simulink model "CubeSat_Simulator"  (R2019a)
settings: Solver=ode4  StartTime=0.0  StopTime=54000  FixedStep=0.1  RelTol=1e-5
model workspace: external: MATLAB File C:\Users\Heyang Zhang\OneDrive\02_Education\01_Undergraduate\02_Capstone\Killick-1 CubeSat\05_Technical\01_Simulation\01_Killick1\Simscape\Killick1_simScape_DataFile.m (data not in the file)
values from neighbouring files (symbols this model uses):
  a_desired = 0.35    [CubeSat_Parameter.m]
  D_distri = G_s.'* inv(G_s * G_s.')    [CubeSat_Parameter.m]
  G_s = [-cos(a_inc)*sin(b_rot)  -cos(a_inc)*cos(b_rot)   cos(a_inc)*sin(b_rot)  cos(a_inc)*cos(b_rot) ... (first row only)    [CubeSat_Parameter.m]
  I_rw = I_s - sum_rw    [CubeSat_Parameter.m]
  I_w = [3500E-9  3500E-9  3500E-9  3500E-9 ... (first row only)    [CubeSat_Parameter.m]
  Kc = [eye(3).*[2.5;2.5;2.5]  eye(3).*[5;5;5]]    [CubeSat_Parameter.m]
  Ki = [eye(3).*[1.2 1.2 1.2]  eye(3).*[3;3;3]]    [CubeSat_Parameter.m]
  Kw_d = 0.4    [CubeSat_Parameter.m]
  Kw_i = 0.1    [CubeSat_Parameter.m]
  Kw_p = 0.4    [CubeSat_Parameter.m]
  OMEGA_0 = [0;0;0]    [CubeSat_Parameter.m]
  quat_0 = eul2quat(eulr_0).'    [CubeSat_Parameter.m]
  SatMass = 3.5    [CubeSat_Parameter.m]
  tau_sat_mt = 1e-3    (= 0.001)    [CubeSat_Parameter.m]
  tau_sat_rw = 5e-3    (= 0.005)    [CubeSat_Parameter.m]
  w_desired = 0.35    [CubeSat_Parameter.m]
  w_rw_ref = [0;0;-0;-0]    [CubeSat_Parameter.m]
undefined symbols (not defined in the file or in its folder): Earth, IAU, km, Kp, Kv, s, WGS84
libraries: sharedutil x19, aerolibutil x18, dspmathops x18, sharedtransform x13, simulink_extras x8, aerolibtransform2 x5, simulink x5, asbCubeSatBlockLib x5, aerolibconvert2 x3, dsparch4 x3, ADCS_lib x2, aerolibcelestial x2
(part 2 of 3)

== system CubeSat_Simulator/CubeSat Hardware/Vehicle Dynamics/Orbital ==
  ExtForce_eci : Inport
  Gain : Gain  Gain=1/SatMass
  Initial Position : Constant  Value=[6778100;0;0]
  Initial Velocity : Constant  Value=[0;5444;5444]
  "Integrator, Second-Order" : SecondOrderIntegrator  ICSourceX=external  ICSourceDXDT=external
  Out Bus Element2 : Outport  PortName=SatStateOrbt  Element=x_eci
  Out Bus Element1 : Outport  PortName=SatStateOrbt  Element=v_eci
  Out Bus Element3 : Outport  PortName=SatStateOrbt  Element=a_eci
  wires:
  Gain/1 -> Out Bus Element3/1, "Integrator, Second-Order"/1
  ExtForce_eci/1 -> Gain/1
  "Integrator, Second-Order"/1 -> Out Bus Element2/1
  "Integrator, Second-Order"/2 -> Out Bus Element1/1
  Initial Velocity/1 -> "Integrator, Second-Order"/3
  Initial Position/1 -> "Integrator, Second-Order"/2

== system CubeSat_Simulator/Environment/Earth Rotation Planet Position/Celestrial Body Position ==
  JulianDate : Inport
  Length Conversion : aerolibconvert2/Length Conversion  IU=km  OU=m
  Length Conversion1 : aerolibconvert2/Length Conversion  IU=km  OU=m
  Moon Position_ECI : aerolibcelestial/Planetary Ephemeris  kmflag=km,km/s  epochflag=Julian date  de=DE405  nCenter=Earth  nTarget=Moon  errorflag=Error  velflag=off
      settings: SourceProductName=Aerospace Blockset  SourceProductBaseCode=AE
  Sun Position_ECI : aerolibcelestial/Planetary Ephemeris  kmflag=km,km/s  epochflag=Julian date  de=DE405  nCenter=Earth  nTarget=Sun  errorflag=Error  velflag=off
      settings: SourceProductName=Aerospace Blockset  SourceProductBaseCode=AE
  x_sun_eci : Outport
  x_moon_eci : Outport  Port=2
  wires:
  Sun Position_ECI/1 -> Length Conversion/1
  JulianDate/1 -> Moon Position_ECI/1, Sun Position_ECI/1
  Moon Position_ECI/1 -> Length Conversion1/1
  Length Conversion/1 -> x_sun_eci/1  "x_sun_eci"
  Length Conversion1/1 -> x_moon_eci/1  "x_moon_eci"

== system CubeSat_Simulator/Environment/Earth Rotation Planet Position/Earth Rotation  ==
  SimTime : Inport
  Direction Cosine Matrix to Quaternions : sharedtransform/Direction Cosine Matrix  to Quaternions  aMode=0  action=None  tolerance=eps(2)
      settings: SourceProductName=Aerospace Blockset  SourceProductBaseCode=AE
  Direction Cosine Matrix to Quaternions1 : sharedtransform/Direction Cosine Matrix  to Quaternions  aMode=0  action=None  tolerance=eps(2)
      settings: SourceProductName=Aerospace Blockset  SourceProductBaseCode=AE
  ECI to ECEF DCM : aerolibtransform2/Direction Cosine Matrix ECI to ECEF  red=IAU-2000/2006  year=2019  month=July  day=1  hour=0  min=0  sec=0  deltaT=Sec  errorflag=Error  extraparamflag=off
      settings: AttributesFormatString=%<red>  SourceProductName=Aerospace Blockset  SourceProductBaseCode=AE
  Transpose : Math  Operator=transpose  SaturateOnIntegerOverflow=on
  q_eci2ecef : Outport
  q_ecef2eci : Outport  Port=2
  wires:
  Transpose/1 -> Direction Cosine Matrix to Quaternions1/1
  Direction Cosine Matrix to Quaternions1/1 -> q_ecef2eci/1
  Direction Cosine Matrix to Quaternions/1 -> q_eci2ecef/1
  ECI to ECEF DCM/1 -> Direction Cosine Matrix to Quaternions/1, Transpose/1
  SimTime/1 -> ECI to ECEF DCM/1

== system CubeSat_Simulator/Environment/External Force and Torque/Earth Gravity Pull ==
  x_ecef : Inport
  Gain : Gain  Gain=SatMass
  Spherical Harmonic Gravity Model : aerolibgravity2/Spherical Harmonic Gravity Model  units=Metric (MKS)  degree=120  action=Warning  ptype=EGM2008  datafile='aerogmm2b.mat'
      settings: SourceProductName=Aerospace Blockset  SourceProductBaseCode=AE
  f_grav_ecef : Outport
  wires:
  Spherical Harmonic Gravity Model/1 -> Gain/1
  Gain/1 -> f_grav_ecef/1
  x_ecef/1 -> Spherical Harmonic Gravity Model/1

== system CubeSat_Simulator/Environment/External Force and Torque/Exp Decay Air Density ==
  h (m) : Inport
  2-D Lookup Table : Lookup_n-D  BreakpointsForDimension1=[12.5 27.5:5:97.5 105:10:170 190 225:50:475 550:100:950]  BreakpointsForDimension2=[1:3]  Table=[0 1.225 8.44; 25 3.899e-2 6.49; 30 1.774e-2 6.75; 35 8.279e-3 7.07; 40 3.972e-3 7.47; 45 1.995e-3 7.83; 50 1.057e-3 7.95; 55 5.821e-4 7.73; 60 3.206e-4 7.29; 65 1.718e-4 6.81; 70 8.770e-5 6.33; 75 4.178e-5 6; 80 1.905e-5 5.7; 85 8.337e-6 5.41; 90 3.396e-6 5.38; 95 1.343e-6 5.74; 100 5.297e-7 6.15; 110 9.661e-8 8.06; 120 2.438e-8 11.6; 130 8.484e-9 16.1; 140 3.845e-9 20.6; 150 2.07e-9 24.6; 160 1.224e-9 26.3; 180 5.464e-10 33.2; 200 2.789e-10 38.5; 250 7.248e-11 46.9; 300 2.418e-11 52.5; 350 9.158e-12 56.4; 400 3.725e-12 59.4; 450 1.585e-12 62.2; 500 6.967e-13 65.8; 600 1.454e-13 79; 700 3.614e-14 109; 800 1.17e-14 164; 900 5.245e-15 225]  InternalRulePriority=Speed  RndMeth=Simplest  InputSameDT=on
  2-D Lookup Table1 : Lookup_n-D  BreakpointsForDimension1=[12.5 27.5:5:97.5 105:10:170 190 225:50:475 550:100:950]  BreakpointsForDimension2=[1:3]  Table=[0 1.225 8.44; 25 3.899e-2 6.49; 30 1.774e-2 6.75; 35 8.279e-3 7.07; 40 3.972e-3 7.47; 45 1.995e-3 7.83; 50 1.057e-3 7.95; 55 5.821e-4 7.73; 60 3.206e-4 7.29; 65 1.718e-4 6.81; 70 8.770e-5 6.33; 75 4.178e-5 6; 80 1.905e-5 5.7; 85 8.337e-6 5.41; 90 3.396e-6 5.38; 95 1.343e-6 5.74; 100 5.297e-7 6.15; 110 9.661e-8 8.06; 120 2.438e-8 11.6; 130 8.484e-9 16.1; 140 3.845e-9 20.6; 150 2.07e-9 24.6; 160 1.224e-9 26.3; 180 5.464e-10 33.2; 200 2.789e-10 38.5; 250 7.248e-11 46.9; 300 2.418e-11 52.5; 350 9.158e-12 56.4; 400 3.725e-12 59.4; 450 1.585e-12 62.2; 500 6.967e-13 65.8; 600 1.454e-13 79; 700 3.614e-14 109; 800 1.17e-14 164; 900 5.245e-15 225]  InternalRulePriority=Speed  RndMeth=Simplest  InputSameDT=on
  2-D Lookup Table2 : Lookup_n-D  BreakpointsForDimension1=[12.5 27.5:5:97.5 105:10:170 190 225:50:475 550:100:950]  BreakpointsForDimension2=[1:3]  Table=[0 1.225 8.44; 25 3.899e-2 6.49; 30 1.774e-2 6.75; 35 8.279e-3 7.07; 40 3.972e-3 7.47; 45 1.995e-3 7.83; 50 1.057e-3 7.95; 55 5.821e-4 7.73; 60 3.206e-4 7.29; 65 1.718e-4 6.81; 70 8.770e-5 6.33; 75 4.178e-5 6; 80 1.905e-5 5.7; 85 8.337e-6 5.41; 90 3.396e-6 5.38; 95 1.343e-6 5.74; 100 5.297e-7 6.15; 110 9.661e-8 8.06; 120 2.438e-8 11.6; 130 8.484e-9 16.1; 140 3.845e-9 20.6; 150 2.07e-9 24.6; 160 1.224e-9 26.3; 180 5.464e-10 33.2; 200 2.789e-10 38.5; 250 7.248e-11 46.9; 300 2.418e-11 52.5; 350 9.158e-12 56.4; 400 3.725e-12 59.4; 450 1.585e-12 62.2; 500 6.967e-13 65.8; 600 1.454e-13 79; 700 3.614e-14 109; 800 1.17e-14 164; 900 5.245e-15 225]  InternalRulePriority=Speed  RndMeth=Simplest  InputSameDT=on
  Index: H [km] : Constant  Value=3
  Index: h_0 [km] : Constant
  Index: rho_0 [kg/m3] : Constant  Value=2
  MATLAB Function3 : MATLAB Function  TreatAsAtomicUnit=on
  Multiply : Gain  Gain=1/1000
  rho (kg/m3) : Outport
  wires:
  Multiply/1 -> 2-D Lookup Table1/1, 2-D Lookup Table/1, 2-D Lookup Table2/1, MATLAB Function3/1(h)
  2-D Lookup Table/1 -> MATLAB Function3/2(h_0)
  2-D Lookup Table2/1 -> MATLAB Function3/4(H)
  Index: rho_0 [kg/m3]/1 -> 2-D Lookup Table1/2
  2-D Lookup Table1/1 -> MATLAB Function3/3(rho_0)
  h (m)/1 -> Multiply/1
  Index: h_0 [km]/1 -> 2-D Lookup Table/2
  Index: H [km]/1 -> 2-D Lookup Table2/2
  MATLAB Function3/1(rho) -> rho (kg/m3)/1

== system CubeSat_Simulator/Environment/External Force and Torque/q to w ==
  q : Inport
  Derivative : Derivative
  Product : Product
  Quaternion to Spatial Rotation : Subsystem
  w : Outport
  wires:
  q/1 -> Quaternion to Spatial Rotation/1(q)
  Derivative/1 -> Product/1
  Product/1 -> w/1
  Quaternion to Spatial Rotation/1(PRA) -> Derivative/1
  Quaternion to Spatial Rotation/2(PRV) -> Product/2  "ehat"

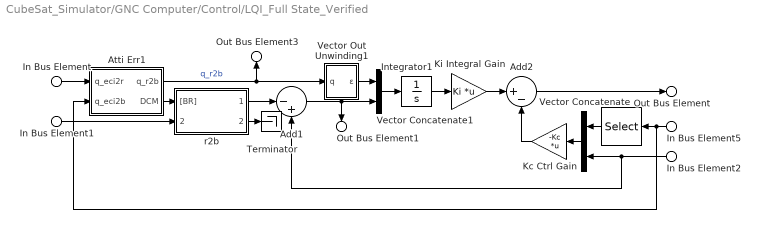
== system CubeSat_Simulator/GNC Computer/Control/LQI_Full State_Verified ==
  In Bus Element : Inport  PortName=GdnIn  Element=q_eci2ref
  In Bus Element1 : Inport  PortName=GdnIn  Element=r_w_r/n
  In Bus Element5 : Inport  Port=2  PortName=NavIn  Element=q_eci2body
  In Bus Element2 : Inport  Port=2  PortName=NavIn  Element=b_w_b/n
  " " : Selector  InputPortWidth=4  IndexOptions=Index vector (dialog)  Indices=[2 3 4]  OutputSizes=1
  Add1 : Sum  Inputs=|-+
  Add2 : Sum  Inputs=|+-
  Atti Err1 : Subsystem
  Integrator1 : Integrator
  Kc Ctrl Gain : Gain  Gain=-Kc  Multiplication=Matrix(K*u)
  Ki Integral Gain : Gain  Gain=Ki  Multiplication=Matrix(K*u)
  Terminator : Terminator
  Vector Concatenate : Concatenate
  Vector Concatenate1 : Concatenate
  Vector Out Unwinding1 : Subsystem
  r2b : Subsystem
  Out Bus Element : Outport  PortName=ACCmd  Element=b_t_total
  Out Bus Element3 : Outport  Port=2  PortName=ErrData  Element=q_r2b
  Out Bus Element1 : Outport  Port=2  PortName=ErrData  Element=deltaw_b/r
  wires:
  Vector Concatenate1/1 -> Integrator1/1
  Vector Out Unwinding1/1(ε) -> Vector Concatenate1/1
  Vector Concatenate/1 -> Kc Ctrl Gain/1
  " "/1 -> Vector Concatenate/1
  Integrator1/1 -> Ki Integral Gain/1
  Add2/1 -> Out Bus Element/1
  Kc Ctrl Gain/1 -> Add2/2
  Ki Integral Gain/1 -> Add2/1
  r2b/2(b_a_r/n) -> Terminator/1
  r2b/1(b_w_r/n) -> Add1/1
  In Bus Element2/1 -> Add1/2, Vector Concatenate/2
  In Bus Element/1 -> Atti Err1/1(q_eci2r)
  Atti Err1/2(DCM) -> r2b/1("[BR]")
  In Bus Element5/1 -> Atti Err1/2(q_eci2b), " "/1
  Atti Err1/1(q_r2b) -> Vector Out Unwinding1/1(q), Out Bus Element3/1  "q_r2b"
  Add1/1 -> Vector Concatenate1/2, Out Bus Element1/1
  In Bus Element1/1 -> r2b/2(r_w_r/n)

== system CubeSat_Simulator/GNC Computer/Control/Momentum Management1 ==
  ACCmd : Inport
  w_rw : Inport  Port=2
  Add : Sum  Inputs=|++
  Bus Creator : BusCreator  Inputs=2
  G_s : Gain  Gain=G_s  Multiplication=Matrix(K*u)
  de-spin torq : Subsystem
  Out Bus Element : Outport  PortName=MMCmd  Element=MMTorqCmd
  wires:
  Bus Creator/1 -> Out Bus Element/1
  ACCmd/1 -> Add/1
  G_s/1 -> Add/2, Bus Creator/2  "b_t_cmd_mtc"
  Add/1 -> Bus Creator/1  "b_t_cmd_rwc"
  w_rw/1 -> de-spin torq/1(w_rw)
  de-spin torq/1(u_despin) -> G_s/1

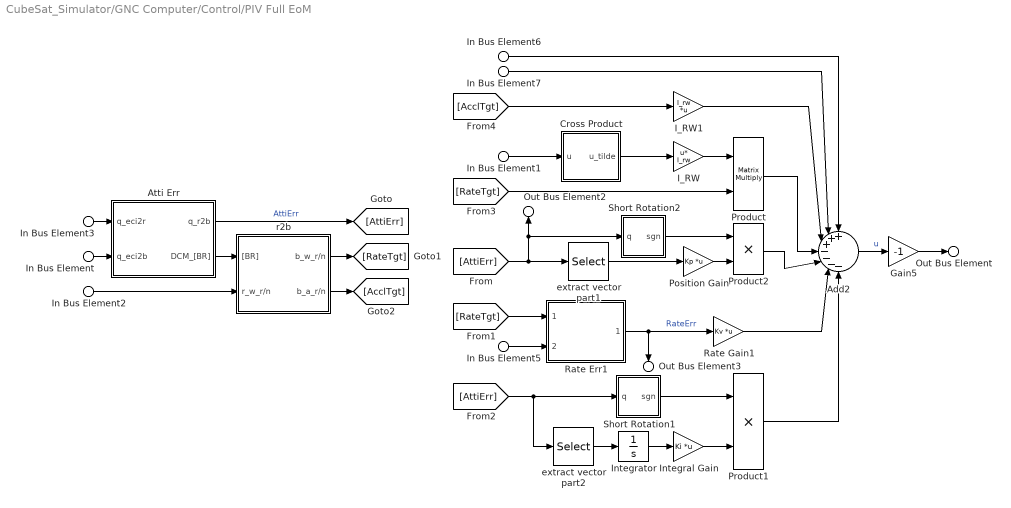
== system CubeSat_Simulator/GNC Computer/Control/PIV Full EoM ==
  In Bus Element3 : Inport  PortName=GdnIn  Element=q_eci2ref
  In Bus Element2 : Inport  PortName=GdnIn  Element=r_w_r/n
  In Bus Element : Inport  Port=2  PortName=NavIn  Element=q_eci2body
  In Bus Element5 : Inport  Port=2  PortName=NavIn  Element=b_w_b/n
  In Bus Element1 : Inport  Port=2  PortName=NavIn  Element=b_w_b/n
  In Bus Element6 : Inport  Port=2  PortName=NavIn  Element=gyroscopic
  In Bus Element7 : Inport  Port=2  PortName=NavIn  Element=momentum
  Add2 : Sum  Inputs=+++----
  Atti Err : Subsystem
  Cross Product : MATLAB Function  TreatAsAtomicUnit=on
  Gain5 : Gain  Gain=-1
  I_RW : Gain  Gain=I_rw  Multiplication=Matrix(u*K)
  I_RW1 : Gain  Gain=I_rw  Multiplication=Matrix(K*u)
  Integral Gain : Gain  Gain=Ki  Multiplication=Matrix(K*u)
  Integrator : Integrator
  Position Gain : Gain  Gain=Kp  Multiplication=Matrix(K*u)
  Product : Product  Multiplication=Matrix(*)
  Product1 : Product
  Product2 : Product
  Rate Err1 : Subsystem
  Rate Gain1 : Gain  Gain=Kv  Multiplication=Matrix(K*u)
  Short Rotation1 : Subsystem
  Short Rotation2 : Subsystem
  extract vector part1 : Selector  InputPortWidth=4  IndexOptions=Index vector (dialog)  Indices=[2 3 4]  OutputSizes=1
  extract vector part2 : Selector  InputPortWidth=4  IndexOptions=Index vector (dialog)  Indices=[2 3 4]  OutputSizes=1
  r2b : Subsystem
  Out Bus Element : Outport  PortName=ACCmd  Element=b_t_total
  Out Bus Element3 : Outport  Port=2  PortName=ErrData  Element=deltaw_b/r
  Out Bus Element2 : Outport  Port=2  PortName=ErrData  Element=q_r2b
  wires:
  Rate Gain1/1 -> Add2/6
  In Bus Element6/1 -> Add2/1
  In Bus Element7/1 -> Add2/2
  I_RW1/1 -> Add2/3
  Product/1 -> Add2/4
  Product2/1 -> Add2/5
  Product1/1 -> Add2/7
  [AcclTgt] -> I_RW1/1
  [RateTgt] -> Product/2
  extract vector part1/1 -> Position Gain/1
  [AttiErr] -> extract vector part1/1, Out Bus Element2/1, Short Rotation2/1(q)
  Short Rotation2/1(sgn) -> Product2/1
  Position Gain/1 -> Product2/2
  Atti Err/1(q_r2b) -> [AttiErr]  "AttiErr"
  In Bus Element2/1 -> r2b/2(r_w_r/n)
  r2b/2(b_a_r/n) -> [AcclTgt]
  Add2/1 -> Gain5/1  "u"
  Gain5/1 -> Out Bus Element/1
  Rate Err1/1(b_deltaw_b/r) -> Out Bus Element3/1, Rate Gain1/1  "RateErr"
  In Bus Element5/1 -> Rate Err1/2(b_w_b/n)
  In Bus Element3/1 -> Atti Err/1(q_eci2r)
  r2b/1(b_w_r/n) -> [RateTgt]
  Atti Err/2(DCM_[BR]) -> r2b/1("[BR]")
  Integral Gain/1 -> Product1/2
  Short Rotation1/1(sgn) -> Product1/1
  [AttiErr] -> extract vector part2/1, Short Rotation1/1(q)
  Integrator/1 -> Integral Gain/1
  extract vector part2/1 -> Integrator/1
  [RateTgt] -> Rate Err1/1(b_w_r/n)
  Cross Product/1(u_tilde) -> I_RW/1
  In Bus Element1/1 -> Cross Product/1(u)
  I_RW/1 -> Product/1
  In Bus Element/1 -> Atti Err/2(q_eci2b)

== system CubeSat_Simulator/GNC Computer/Guidance/Inertial Pointing ==
  Degrees to Radians : simulink_extras/Transformations/Degrees to Radians
  Spatial Rotation to Quaternion : Subsystem
  Step1 : Step  Time=10  After=0  SampleTime=0
  axis : Constant  Value=[1;1;1]
  q_eci2iner : Outport
  wires:
  axis/1 -> Spatial Rotation to Quaternion/2(PRV)
  Degrees to Radians/1 -> Spatial Rotation to Quaternion/1(PRA)
  Step1/1 -> Degrees to Radians/1
  Spatial Rotation to Quaternion/1(q) -> q_eci2iner/1

== system CubeSat_Simulator/GNC Computer/Guidance/Nadir Pointing ==
  NadirBias : Inport
  SensorIn : Inport  Port=2
  Align Body Axis : Subsystem
  Apply Orientation Bias : Subsystem
  Calculate Hill Frame : Subsystem
  q_eci2nadr : Outport
  wires:
  Align Body Axis/1(q_eci2ndir) -> Apply Orientation Bias/1(q_eci2ndir)
  Apply Orientation Bias/1(q_eci2imag) -> q_eci2nadr/1
  NadirBias/1 -> Apply Orientation Bias/2(NadirBias)
  SensorIn/1 -> Calculate Hill Frame/1(SensorIn)
  Calculate Hill Frame/1(q_eci2hill) -> Align Body Axis/1(q_eci2hill)

== system CubeSat_Simulator/GNC Computer/Guidance/Orbital Velocity Frame (Visualization Only) ==
  In Bus Element1 : Inport  PortName=SensorIn  Element=x_eci
  In Bus Element2 : Inport  PortName=SensorIn  Element=v_eci
  3x3 Cross Product2 : sharedutil/3x3 Cross Product  aMode=aMode
      settings: SourceProductBaseCode=AE
  3x3 Cross Product3 : sharedutil/3x3 Cross Product  aMode=aMode
      settings: SourceProductBaseCode=AE
  Direction Cosine Matrix to Quaternions : sharedtransform/Direction Cosine Matrix  to Quaternions  aMode=0  action=None  tolerance=eps(2)
      settings: SourceProductName=Aerospace Blockset  SourceProductBaseCode=AE
  Gain : Gain  Gain=-1
  Normalization3 : dspmathops/Normalization  NormType=2-norm  Bias=1e-10  NormOver=Each column  Dimension=1  roundingMode=Floor  overflowMode=off  accumDataTypeStr=Inherit: Same as product output  accumLastDataTypeStr=Inherit: Same as product output  outputDataTypeStr=Inherit: Same as product output  outputMin=[]  outputMax=[]  outputLastDataTypeStr=Inherit: Same as product output
      settings: SourceProductName=DSP System Toolbox
  Normalization4 : dspmathops/Normalization  NormType=2-norm  Bias=1e-10  NormOver=Each column  Dimension=1  roundingMode=Floor  overflowMode=off  accumDataTypeStr=Inherit: Same as product output  accumLastDataTypeStr=Inherit: Same as product output  outputDataTypeStr=Inherit: Same as product output  outputMin=[]  outputMax=[]  outputLastDataTypeStr=Inherit: Same as product output
      settings: SourceProductName=DSP System Toolbox
  Quaternion Normalize : sharedutil/Quaternion Normalize  aMode=aMode
      settings: SourceProductName=Aerospace Blockset  SourceProductBaseCode=AE
  Transpose : Math  Operator=transpose  SaturateOnIntegerOverflow=on
  Transpose1 : Math  Operator=transpose  SaturateOnIntegerOverflow=on
  Transpose2 : Math  Operator=transpose  SaturateOnIntegerOverflow=on
  Vector Concatenate : Concatenate  NumInputs=3  Mode=Multidimensional array
  q_eci2velo : Outport
  wires:
  Direction Cosine Matrix to Quaternions/1 -> Quaternion Normalize/1
  Transpose1/1 -> Vector Concatenate/3
  Vector Concatenate/1 -> Direction Cosine Matrix to Quaternions/1
  Transpose2/1 -> Vector Concatenate/2
  Transpose/1 -> Vector Concatenate/1
  In Bus Element2/1 -> Normalization3/1
  Normalization3/1 -> Gain/1
  Gain/1 -> 3x3 Cross Product3/1, Transpose/1, 3x3 Cross Product2/2
  In Bus Element1/1 -> Normalization4/1
  Normalization4/1 -> 3x3 Cross Product2/1
  3x3 Cross Product2/1 -> Transpose2/1, 3x3 Cross Product3/2
  3x3 Cross Product3/1 -> Transpose1/1
  Quaternion Normalize/1 -> q_eci2velo/1

== system CubeSat_Simulator/GNC Computer/Guidance/Sun Tracking ==
  SunBias : Inport
  In Bus Element1 : Inport  Port=2  PortName=SensorIn  Element=x_eci
  In Bus Element : Inport  Port=3  PortName=EnvState  Element=Celestrial.x_sun_eci
  Add1 : Sum  Inputs=+-
  Attitude Bias : Subsystem
  Check Parallel : asbCubeSatBlockLib/Axes Transformations/Attitude Conversion/Check Parallel  SystemSampleTime=-1
  Compare To Zero1 : simulink/Logic and Bit Operations/Compare To Zero  relop=~=  OutDataTypeStr=boolean
  Compute Sun Frame : Subsystem
  ECI X Axis : Constant  Value=[1;0;0]
  ECI Z Axis : Constant  Value=[0;0;1]
  If Sun Directly Above ECI : asbCubeSatBlockLib/Axes Transformations/Attitude Conversion/Quaternion between r_a and r_b  SystemSampleTime=-1
  Switch 1 走上 0 走下 : Switch  Criteria=u2 ~= 0
  q_eci2sun : Outport
  wires:
  Add1/1 -> If Sun Directly Above ECI/2, Check Parallel/1, Compute Sun Frame/1(FirstRefECI)
  ECI Z Axis/1 -> Check Parallel/2, Compute Sun Frame/2(SecondRefECI)
  Compute Sun Frame/1(q_eci2sun) -> Switch 1 走上 0 走下/3
  In Bus Element/1 -> Add1/1
  In Bus Element1/1 -> Add1/2
  ECI X Axis/1 -> If Sun Directly Above ECI/1
  If Sun Directly Above ECI/1 -> Switch 1 走上 0 走下/1
  Check Parallel/1 -> Compare To Zero1/1
  Compare To Zero1/1 -> Switch 1 走上 0 走下/2
  Switch 1 走上 0 走下/1 -> Attitude Bias/1(q Input)
  Attitude Bias/1("\tq Output") -> q_eci2sun/1
  SunBias/1 -> Attitude Bias/2(EulerBias)

== system CubeSat_Simulator/GNC Computer/Guidance/Target Tracking ==
  TargetLLA : Inport
  TargetBias : Inport  Port=2
  In Bus Element1 : Inport  Port=3  PortName=SensorIn  Element=x_eci
  In Bus Element : Inport  Port=4  PortName=EnvState  Element=Celestrial.q_ecef2eci
  Add1 : Sum  Inputs=|+-
  Attitude Bias : Subsystem
  Check Parallel : asbCubeSatBlockLib/Axes Transformations/Attitude Conversion/Check Parallel  SystemSampleTime=-1
  Compare To Zero1 : simulink/Logic and Bit Operations/Compare To Zero  relop=~=  OutDataTypeStr=boolean
  Compute Sun Frame : Subsystem
  Demux : Demux  Outputs=3
  ECI X Axis : Constant  Value=[1;0;0]
  ECI Z Axis : Constant  Value=[0;0;1]
  If Sun Directly Above ECI : asbCubeSatBlockLib/Axes Transformations/Attitude Conversion/Quaternion between r_a and r_b  SystemSampleTime=-1
  "LLA to ECEF Position " : aerolibtransform2/LLA to ECEF Position  units=Metric (MKS)  ptype=Earth (WGS84)  F=1/298.257223563  R=6378137
      settings: SourceProductName=Aerospace Blockset  SourceProductBaseCode=AE
  Mux : Mux  Inputs=2
  Switch 1 走上 0 走下 : Switch  Criteria=u2 ~= 0
  Target Position ECEF to ECI : aerolibutil/Quaternion Rotation
  q_eci2lla : Outport
  tag scope: TgtPos_eci=global
  wires:
  Attitude Bias/1("\tq Output") -> q_eci2lla/1
  In Bus Element/1 -> Target Position ECEF to ECI/1
  "LLA to ECEF Position "/1 -> Target Position ECEF to ECI/2
  Demux/1 -> Mux/1
  Demux/2 -> Mux/2
  Mux/1 -> "LLA to ECEF Position "/1
  TargetLLA/1 -> Demux/1
  Demux/3 -> "LLA to ECEF Position "/2
  In Bus Element1/1 -> Add1/1
  Target Position ECEF to ECI/1 -> Add1/2
  Add1/1 -> Compute Sun Frame/1(FirstRefECI), [TgtPos_eci], Check Parallel/1, If Sun Directly Above ECI/2  "TgtPos_eci"
  If Sun Directly Above ECI/1 -> Switch 1 走上 0 走下/1
  TargetBias/1 -> Attitude Bias/2(EulerBias)
  Check Parallel/1 -> Compare To Zero1/1
  Switch 1 走上 0 走下/1 -> Attitude Bias/1(q Input)
  ECI X Axis/1 -> If Sun Directly Above ECI/1
  Compare To Zero1/1 -> Switch 1 走上 0 走下/2
  ECI Z Axis/1 -> Check Parallel/2, Compute Sun Frame/2(SecondRefECI)
  Compute Sun Frame/1(q_eci2sun) -> Switch 1 走上 0 走下/3

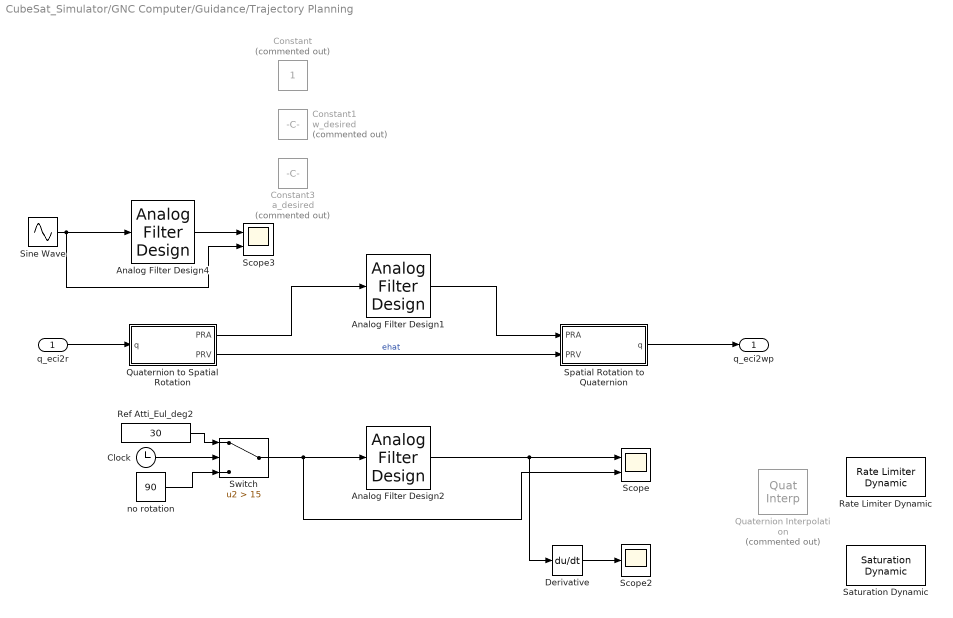
== system CubeSat_Simulator/GNC Computer/Guidance/Trajectory Planning ==
  q_eci2r : Inport
  Analog Filter Design1 : dsparch4/Analog Filter Design  method=Bessel  filttype=Lowpass  N=10  Wlo=0.1  Whi=80  Rp=2  Rs=40
  Analog Filter Design2 : dsparch4/Analog Filter Design  method=Bessel  filttype=Lowpass  N=10  Wlo=0.5  Whi=80  Rp=2  Rs=40
  Analog Filter Design4 : dsparch4/Analog Filter Design  method=Bessel  filttype=Lowpass  N=10  Wlo=0.1  Whi=80  Rp=2  Rs=40
  Clock : Clock
  Constant : Constant  Commented=on
  Constant1 : Constant  Commented=on  Value=w_desired
  Constant3 : Constant  Commented=on  Value=a_desired
  Derivative : Derivative
  Quaternion Interpolation : QuatInterp  Commented=on
  Quaternion to Spatial Rotation : Subsystem
  Rate Limiter Dynamic : simulink/Discontinuities/Rate Limiter Dynamic
      settings: SourceProductName=Simulink
  Ref Atti_Eul_deg2 : Constant  Value=30
  Saturation Dynamic : simulink/Discontinuities/Saturation Dynamic  OutMin=[]  OutMax=[]  OutDataTypeStr=Inherit: Same as second input  OutDataType=fixdt(1, 16)  OutScaling=2^-10  DoSatur=off
  Scope : Scope  NumInputPorts=2
  Scope2 : Scope
  Scope3 : Scope  NumInputPorts=2
  Sine Wave : Sin  Amplitude=89  Frequency=0.00628  SampleTime=0
  Spatial Rotation to Quaternion : Subsystem
  Switch : Switch  Criteria=u2 > Threshold  Threshold=15
  no rotation : Constant  Value=90
  q_eci2wp : Outport
  wires:
  q_eci2r/1 -> Quaternion to Spatial Rotation/1(q)
  Quaternion to Spatial Rotation/2(PRV) -> Spatial Rotation to Quaternion/2(PRV)  "ehat"
  Clock/1 -> Switch/2
  no rotation/1 -> Switch/3
  Switch/1 -> Analog Filter Design2/1, Scope/2
  Derivative/1 -> Scope2/1
  Ref Atti_Eul_deg2/1 -> Switch/1
  Quaternion to Spatial Rotation/1(PRA) -> Analog Filter Design1/1
  Analog Filter Design1/1 -> Spatial Rotation to Quaternion/1(PRA)
  Spatial Rotation to Quaternion/1(q) -> q_eci2wp/1
  Analog Filter Design2/1 -> Derivative/1, Scope/1
  Sine Wave/1 -> Scope3/2, Analog Filter Design4/1
  Analog Filter Design4/1 -> Scope3/1

== system CubeSat_Simulator/GNC Computer/Guidance/Trapzodial Velocity Profile ==
  p_desired : Inport
  v_desired : Inport  Port=2
  a_desired : Inport  Port=3
  Display6 : Display  Commented=on
  MATLAB Function : MATLAB Function  Commented=on  TreatAsAtomicUnit=on
      mask init:
      | w = 0;
  MATLAB Function1 : MATLAB Function  Commented=on  TreatAsAtomicUnit=on
      mask init:
      | w = 0;
  Scope : Scope  Commented=on
  key time stamp : Subsystem
  wires:
  p_desired/1 -> key time stamp/1(p_input)
  a_desired/1 -> key time stamp/3(a_input)
  v_desired/1 -> key time stamp/2(v_input)
  MATLAB Function/1(p_traj) -> Scope/1
  key time stamp/2(v) -> MATLAB Function1/1(v)
  key time stamp/3(a) -> MATLAB Function1/2(a)
  key time stamp/4(t_acc) -> MATLAB Function1/3(T1)
  MATLAB Function1/1(y) -> Display6/1

== system CubeSat_Simulator/CubeSat Hardware/Attitude Actuator/Reaction Wheel Cluster/RW 1 ==
  OMEGA : Inport
  ALPHA : Inport  Port=2
  u_s_1 : Inport  Port=3
  G_s : Gain  Gain=G_s(:,1).'  Multiplication=Matrix(K*u)
  Gain : Gain  Gain=1/I_w(1,1)
  Gain1 : Gain  Gain=G_s(:,1).'  Multiplication=Matrix(K*u)
  I_w : Gain  Gain=I_w(1,1)
  Integrator : Integrator
  Sum : Sum  Inputs=+-
  Sum1 : Sum
  h_w_1 : Outport
  omega_w_1 : Outport  Port=2
  wires:
  Sum/1 -> Integrator/1
  Integrator/1 -> Sum1/2, omega_w_1/1
  u_s_1/1 -> Gain/1
  Gain/1 -> Sum/1
  Gain1/1 -> Sum/2
  ALPHA/1 -> Gain1/1
  Sum1/1 -> I_w/1
  I_w/1 -> h_w_1/1
  G_s/1 -> Sum1/1
  OMEGA/1 -> G_s/1

== system CubeSat_Simulator/CubeSat Hardware/Attitude Actuator/Reaction Wheel Cluster/RW 2 ==
  OMEGA : Inport
  ALPHA : Inport  Port=2
  u_s_2 : Inport  Port=3
  Gain : Gain  Gain=1/I_w(1,2)
  Gain1 : Gain  Gain=G_s(:,2).'  Multiplication=Matrix(K*u)
  Gain2 : Gain  Gain=G_s(:,2).'  Multiplication=Matrix(K*u)
  I_w : Gain  Gain=I_w(1,2)
  Integrator : Integrator
  Sum : Sum  Inputs=+-
  Sum1 : Sum
  h_w_2 : Outport
  omega_w_2 : Outport  Port=2
  wires:
  OMEGA/1 -> Gain2/1
  Gain2/1 -> Sum1/1
  I_w/1 -> h_w_2/1
  Sum1/1 -> I_w/1
  ALPHA/1 -> Gain1/1
  Gain1/1 -> Sum/2
  Gain/1 -> Sum/1
  u_s_2/1 -> Gain/1
  Integrator/1 -> omega_w_2/1, Sum1/2
  Sum/1 -> Integrator/1

== system CubeSat_Simulator/CubeSat Hardware/Attitude Actuator/Reaction Wheel Cluster/RW 3 ==
  OMEGA : Inport
  ALPHA : Inport  Port=2
  u_s_3 : Inport  Port=3
  Gain : Gain  Gain=1/I_w(1,3)
  Gain1 : Gain  Gain=G_s(:,3).'  Multiplication=Matrix(K*u)
  Gain2 : Gain  Gain=G_s(:,3).'  Multiplication=Matrix(K*u)
  I_w : Gain  Gain=I_w(1,3)
  Integrator : Integrator
  Sum : Sum  Inputs=|+-
  Sum1 : Sum  Inputs=|++
  h_w_3 : Outport
  omega_w_3 : Outport  Port=2
  wires:
  Sum/1 -> Integrator/1
  Integrator/1 -> Sum1/2, omega_w_3/1
  u_s_3/1 -> Gain/1
  Gain/1 -> Sum/1
  Gain1/1 -> Sum/2
  ALPHA/1 -> Gain1/1
  Sum1/1 -> I_w/1
  I_w/1 -> h_w_3/1
  Gain2/1 -> Sum1/1
  OMEGA/1 -> Gain2/1

== system CubeSat_Simulator/CubeSat Hardware/Attitude Actuator/Reaction Wheel Cluster/RW 4 ==
  OMEGA : Inport
  ALPHA : Inport  Port=2
  u_s_4 : Inport  Port=3
  Gain : Gain  Gain=1/I_w(1,4)
  Gain1 : Gain  Gain=G_s(:,4).'  Multiplication=Matrix(K*u)
  Gain2 : Gain  Gain=G_s(:,4).'  Multiplication=Matrix(K*u)
  I_w : Gain  Gain=I_w(1,4)
  Integrator : Integrator
  Sum : Sum  Inputs=+-
  Sum1 : Sum
  h_w_4 : Outport
  omega_w_4 : Outport  Port=2
  wires:
  OMEGA/1 -> Gain2/1
  Gain2/1 -> Sum1/1
  I_w/1 -> h_w_4/1
  Sum1/1 -> I_w/1
  ALPHA/1 -> Gain1/1
  Gain1/1 -> Sum/2
  Gain/1 -> Sum/1
  u_s_4/1 -> Gain/1
  Integrator/1 -> omega_w_4/1, Sum1/2
  Sum/1 -> Integrator/1

== system CubeSat_Simulator/CubeSat Hardware/Vehicle Dynamics/Attitude/integrate quaternion ==
  b_w_b/n : Inport
  Constant : Constant  Value=0
  Gain : Gain  Gain=0.5
  Integrator : Integrator  InitialCondition=quat_0
  Quaternion Multiplication : aerolibutil/Quaternion Multiplication
  Quaternion Normalize : sharedutil/Quaternion Normalize  aMode=aMode
      settings: SourceProductName=Aerospace Blockset  SourceProductBaseCode=AE
  Vector Concatenate : Concatenate
  q_eci2b : Outport
  wires:
  Quaternion Multiplication/1 -> Integrator/1
  b_w_b/n/1 -> Vector Concatenate/2
  Integrator/1 -> Quaternion Normalize/1
  Gain/1 -> Quaternion Multiplication/1
  Vector Concatenate/1 -> Quaternion Multiplication/2
  Constant/1 -> Vector Concatenate/1
  Quaternion Normalize/1 -> q_eci2b/1, Gain/1

== system CubeSat_Simulator/Environment/External Force and Torque/q to w/Quaternion to Spatial Rotation ==
  q : Inport
  Constant : Constant  Value=[0;0;0]
  Divide : Product  Inputs=*/
  Gain : Gain  Gain=2
  Normalization : dspmathops/Normalization  NormType=2-norm  Bias=1e-10  NormOver=Each column  Dimension=1  roundingMode=Floor  overflowMode=off  accumDataTypeStr=Inherit: Same as product output  accumLastDataTypeStr=Inherit: Same as product output  outputDataTypeStr=Inherit: Same as product output  outputMin=[]  outputMax=[]  outputLastDataTypeStr=Inherit: Same as product output
      settings: SourceProductName=DSP System Toolbox
  Resolve Division by 0 : Switch  Criteria=u2 ~= 0
  Scalar Part : Selector  InputPortWidth=4  IndexOptions=Index vector (dialog)  Indices=[1]  OutputSizes=1
  Trigonometric Function : Trigonometry  Operator=acos
  Trigonometric Function1 : Trigonometry  OutputSignalType=real
  Vector Part : Selector  InputPortWidth=4  IndexOptions=Index vector (dialog)  Indices=[2 3 4]  OutputSizes=1
  PRA : Outport
  PRV : Outport  Port=2
  wires:
  q/1 -> Scalar Part/1, Vector Part/1
  Scalar Part/1 -> Trigonometric Function/1
  Gain/1 -> PRA/1
  Vector Part/1 -> Divide/1
  Trigonometric Function/1 -> Trigonometric Function1/1, Gain/1
  Trigonometric Function1/1 -> Resolve Division by 0/2, Divide/2
  Normalization/1 -> PRV/1
  Divide/1 -> Resolve Division by 0/1
  Resolve Division by 0/1 -> Normalization/1
  Constant/1 -> Resolve Division by 0/3

== system CubeSat_Simulator/GNC Computer/Control/LQI_Full State_Verified/Atti Err1 ==
  q_eci2r : Inport
  q_eci2b : Inport  Port=2
  Quaternion Inverse1 : aerolibutil/Quaternion Inverse
      settings: SourceProductName=Aerospace Blockset
  Quaternion Multiplication : aerolibutil/Quaternion Multiplication
  "[BR]" : sharedtransform/Quaternions to  Direction Cosine Matrix  aMode=aMode
      settings: SourceProductName=Aerospace Blockset  SourceProductBaseCode=AE
  q_r2b : Outport
  DCM : Outport  Port=2
  wires:
  Quaternion Inverse1/1 -> Quaternion Multiplication/1
  "[BR]"/1 -> DCM/1
  q_eci2r/1 -> Quaternion Multiplication/2
  q_eci2b/1 -> Quaternion Inverse1/1
  Quaternion Multiplication/1 -> "[BR]"/1, q_r2b/1

== system CubeSat_Simulator/GNC Computer/Control/LQI_Full State_Verified/Vector Out Unwinding1 ==
  q : Inport
  Product2 : Product
  Short Rotation : Subsystem
  vector part : Selector  InputPortWidth=4  IndexOptions=Index vector (dialog)  Indices=[2 3 4]  OutputSizes=1
  ε : Outport
  wires:
  Product2/1 -> ε/1
  Short Rotation/1(sgn) -> Product2/1
  q/1 -> Short Rotation/1(q), vector part/1
  vector part/1 -> Product2/2

== system CubeSat_Simulator/GNC Computer/Control/LQI_Full State_Verified/r2b ==
  "[BR]" : Inport
  r_w_r/n : Inport  Port=2
  Derivative : Derivative
  Product : Product  Multiplication=Matrix(*)
  Product1 : Product  Multiplication=Matrix(*)
  b_w_r/n : Outport
  b_a_r/n : Outport  Port=2
  wires:
  Product/1 -> b_w_r/n/1
  Product1/1 -> b_a_r/n/1
  Derivative/1 -> Product1/2  "r_a_r/n"
  "[BR]"/1 -> Product/1, Product1/1
  r_w_r/n/1 -> Derivative/1, Product/2

== system CubeSat_Simulator/GNC Computer/Control/Momentum Management1/de-spin torq ==
  w_rw : Inport
  Add : Sum  Inputs=+-
  Gain : Gain  Gain=-1
  I_w : Gain  Gain=I_w(1,:).'
  PID Controller1 : simulink/Continuous/PID Controller  Controller=PID  Form=Parallel  TimeDomain=Continuous-time  SampleTime=-1  IntegratorMethod=Forward Euler  FilterMethod=Forward Euler  ControllerParametersSource=internal  P=Kw_p  I=Kw_i  D=Kw_d  UseFilter=on  N=10  TunerSelectOption=Transfer Function Based (PID Tuner App)  InitialConditionSource=internal  InitialConditionForIntegrator=0  InitialConditionForFilter=0  DifferentiatorICPrevScaledInput=0  ExternalReset=none  TrackingMode=off  Kt=1  LimitOutput=off  UpperSaturationLimit=tau_sat_mt  LowerSaturationLimit=-tau_sat_mt  LinearizeAsGain=on  AntiWindupMode=clamping  Kb=1  POutMin=[]  POutMax=[]  IOutMin=[]  IOutMax=[]  DOutMin=[]  DOutMax=[]  NOutMin=[]  NOutMax=[]  SumOutMin=[]  SumOutMax=[]  SaturationOutMin=[]  SaturationOutMax=[]  PParamMin=[]  PParamMax=[]  IParamMin=[]  IParamMax=[]  DParamMin=[]  DParamMax=[]  NParamMin=[]  NParamMax=[]  KbParamMin=[]  KbParamMax=[]  KtParamMin=[]  KtParamMax=[]  KbOutMin=[]  KbOutMax=[]  KtOutMin=[]  KtOutMax=[]  IntegratorOutMin=[]  IntegratorOutMax=[]  FilterOutMin=[]  FilterOutMax=[]  SumI1OutMin=[]  SumI1OutMax=[]  SumI2OutMin=[]  SumI2OutMax=[]  SumI3OutMin=[]  SumI3OutMax=[]  SumI4OutMin=[]  SumI4OutMax=[]  SumDOutMin=[]  SumDOutMax=[]  DifferentiatorOutMin=[]  DifferentiatorOutMax=[]  FilterDiffOutCoefMin=[]  FilterDiffOutCoefMax=[]  ReciprocalOutMin=[]  ReciprocalOutMax=[]  SumDenOutMin=[]  SumDenOutMax=[]  SumNumOutMin=[]  SumNumOutMax=[]  DivideOutMin=[]  DivideOutMax=[]  IntegratorContinuousStateAttributes=''  IntegratorStateMustResolveToSignalObject=off  IntegratorRTWStateStorageClass=Auto  FilterContinuousStateAttributes=''  FilterStateMustResolveToSignalObject=off  FilterRTWStateStorageClass=Auto  ParallelPVariant=InternalParameters  IdealPVariant=Disabled  IVariant=InternalParameters  DVariant=InternalParameters  IntegratorVariant=Continuous  SatVariant=Disabled  AWVariant=Passthrough  PCopyVariant=Disabled  TRVariant=Disabled  FdbkBlocksVariant=Forward  IdealPFdbkVariant=Disabled  SatFdbkVariant=Disabled  DerivativeFilterVariant=ContFilter  NVariant=InternalParameters  NCopyVariant=Disabled  FilterICVariant=InternalICsFilter  IntegratorICVariant=InternalICs  ExternalResetVariant=Disabled  TRSumVariant=Passthrough  SumFdbkVariant=Disabled  SumVariant=Sum_PID
  w_rw_ref : Constant  Value=w_rw_ref
  u_despin : Outport
  wires:
  I_w/1 -> PID Controller1/1
  w_rw_ref/1 -> Add/2
  PID Controller1/1 -> Gain/1
  Gain/1 -> u_despin/1
  Add/1 -> I_w/1
  w_rw/1 -> Add/1

== system CubeSat_Simulator/GNC Computer/Control/PIV Full EoM/Atti Err ==
  q_eci2r : Inport
  q_eci2b : Inport  Port=2
  Quaternion Inverse1 : aerolibutil/Quaternion Inverse
      settings: SourceProductName=Aerospace Blockset
  Quaternion Multiplication : aerolibutil/Quaternion Multiplication
  "[BR]" : sharedtransform/Quaternions to  Direction Cosine Matrix  aMode=aMode
      settings: SourceProductName=Aerospace Blockset  SourceProductBaseCode=AE
  q_r2b : Outport
  DCM_[BR] : Outport  Port=2
  wires:
  Quaternion Inverse1/1 -> Quaternion Multiplication/1
  "[BR]"/1 -> DCM_[BR]/1
  q_eci2r/1 -> Quaternion Multiplication/2
  q_eci2b/1 -> Quaternion Inverse1/1
  Quaternion Multiplication/1 -> "[BR]"/1, q_r2b/1

== system CubeSat_Simulator/GNC Computer/Control/PIV Full EoM/Rate Err1 ==
  b_w_r/n : Inport
  b_w_b/n : Inport  Port=2
  Add1 : Sum  Inputs=+-
  b_deltaw_b/r : Outport
  wires:
  Add1/1 -> b_deltaw_b/r/1
  b_w_b/n/1 -> Add1/1
  b_w_r/n/1 -> Add1/2

== system CubeSat_Simulator/GNC Computer/Control/PIV Full EoM/Short Rotation1 ==
  q : Inport
  Gain1 : Gain  Gain=-1
  Sign1 : Signum
  extract scalar part : Selector  InputPortWidth=4  IndexOptions=Index vector (dialog)  Indices=[1]  OutputSizes=1
  sgn : Outport
  wires:
  Gain1/1 -> sgn/1
  Sign1/1 -> Gain1/1
  extract scalar part/1 -> Sign1/1
  q/1 -> extract scalar part/1

== system CubeSat_Simulator/GNC Computer/Control/PIV Full EoM/Short Rotation2 ==
  q : Inport
  Gain1 : Gain  Gain=-1
  Sign1 : Signum
  extract scalar part : Selector  InputPortWidth=4  IndexOptions=Index vector (dialog)  Indices=[1]  OutputSizes=1
  sgn : Outport
  wires:
  q/1 -> extract scalar part/1
  extract scalar part/1 -> Sign1/1
  Sign1/1 -> Gain1/1
  Gain1/1 -> sgn/1

== system CubeSat_Simulator/GNC Computer/Control/PIV Full EoM/r2b ==
  "[BR]" : Inport
  r_w_r/n : Inport  Port=2
  Derivative : Derivative
  Product : Product  Multiplication=Matrix(*)
  Product1 : Product  Multiplication=Matrix(*)
  b_w_r/n : Outport
  b_a_r/n : Outport  Port=2
  wires:
  Product/1 -> b_w_r/n/1
  Product1/1 -> b_a_r/n/1
  Derivative/1 -> Product1/2  "r_a_r/n"
  "[BR]"/1 -> Product/1, Product1/1
  r_w_r/n/1 -> Derivative/1, Product/2

== system CubeSat_Simulator/GNC Computer/Guidance/Inertial Pointing/Spatial Rotation to Quaternion ==
  PRA : Inport
  PRV : Inport  Port=2
  Gain1 : Gain  Gain=0.5
  Mux : Mux  Inputs=2
  Normalization : dspmathops/Normalization  NormType=2-norm  Bias=1e-10  NormOver=Each column  Dimension=1  roundingMode=Floor  overflowMode=off  accumDataTypeStr=Inherit: Same as product output  accumLastDataTypeStr=Inherit: Same as product output  outputDataTypeStr=Inherit: Same as product output  outputMin=[]  outputMax=[]  outputLastDataTypeStr=Inherit: Same as product output
      settings: SourceProductName=DSP System Toolbox
  Product : Product
  Quaternion Normalize : sharedutil/Quaternion Normalize  aMode=aMode
      settings: SourceProductName=Aerospace Blockset  SourceProductBaseCode=AE
  Trigonometric Function2 : Trigonometry  Operator=cos  OutputSignalType=real
  Trigonometric Function3 : Trigonometry  OutputSignalType=real
  q : Outport
  wires:
  PRA/1 -> Gain1/1
  Gain1/1 -> Trigonometric Function3/1, Trigonometric Function2/1
  Trigonometric Function2/1 -> Mux/1
  Trigonometric Function3/1 -> Product/1
  PRV/1 -> Normalization/1
  Product/1 -> Mux/2
  Mux/1 -> Quaternion Normalize/1
  Quaternion Normalize/1 -> q/1
  Normalization/1 -> Product/2

== system CubeSat_Simulator/GNC Computer/Guidance/Nadir Pointing/Align Body Axis ==
  q_eci2hill : Inport
  0;180;-90 : Constant  Value=[0;180;-90]
  Degrees to Radians : simulink_extras/Transformations/Degrees to Radians
  Quaternion Multiplication : aerolibutil/Quaternion Multiplication
  Quaternion Normalize : sharedutil/Quaternion Normalize  aMode=aMode
      settings: SourceProductName=Aerospace Blockset  SourceProductBaseCode=AE
  Rotation Angles to Quaternions : sharedtransform/Rotation Angles to Quaternions  rotationOrder=ZYX  aMode=aMode
      settings: SourceProductName=Aerospace Blockset  SourceProductBaseCode=AE
  q_eci2ndir : Outport
  wires:
  Rotation Angles to Quaternions/1 -> Quaternion Multiplication/2
  q_eci2hill/1 -> Quaternion Multiplication/1
  Degrees to Radians/1 -> Rotation Angles to Quaternions/1
  0;180;-90/1 -> Degrees to Radians/1
  Quaternion Multiplication/1 -> Quaternion Normalize/1
  Quaternion Normalize/1 -> q_eci2ndir/1

== system CubeSat_Simulator/GNC Computer/Guidance/Nadir Pointing/Apply Orientation Bias ==
  q_eci2ndir : Inport
  NadirBias : Inport  Port=2
  Quaternion Multiplication : aerolibutil/Quaternion Multiplication
  Quaternion Normalize : sharedutil/Quaternion Normalize  aMode=aMode
      settings: SourceProductName=Aerospace Blockset  SourceProductBaseCode=AE
  Rotation Angles to Quaternions : sharedtransform/Rotation Angles to Quaternions  rotationOrder=ZYX  aMode=aMode
      settings: SourceProductName=Aerospace Blockset  SourceProductBaseCode=AE
  q_eci2imag : Outport
  wires:
  NadirBias/1 -> Rotation Angles to Quaternions/1
  q_eci2ndir/1 -> Quaternion Multiplication/1
  Rotation Angles to Quaternions/1 -> Quaternion Multiplication/2
  Quaternion Multiplication/1 -> Quaternion Normalize/1
  Quaternion Normalize/1 -> q_eci2imag/1

== system CubeSat_Simulator/GNC Computer/Guidance/Nadir Pointing/Calculate Hill Frame ==
  In Bus Element1 : Inport  PortName=SensorIn  Element=x_eci
  In Bus Element2 : Inport  PortName=SensorIn  Element=v_eci
  3x3 Cross Product : sharedutil/3x3 Cross Product  aMode=aMode
      settings: SourceProductBaseCode=AE
  3x3 Cross Product1 : sharedutil/3x3 Cross Product  aMode=aMode
      settings: SourceProductBaseCode=AE
  Direction Cosine Matrix to Quaternions : sharedtransform/Direction Cosine Matrix  to Quaternions  aMode=0  action=None  tolerance=eps(2)
      settings: SourceProductName=Aerospace Blockset  SourceProductBaseCode=AE
  Normalization1 : dspmathops/Normalization  NormType=2-norm  Bias=1e-10  NormOver=Each column  Dimension=1  roundingMode=Floor  overflowMode=off  accumDataTypeStr=Inherit: Same as product output  accumLastDataTypeStr=Inherit: Same as product output  outputDataTypeStr=Inherit: Same as product output  outputMin=[]  outputMax=[]  outputLastDataTypeStr=Inherit: Same as product output
      settings: SourceProductName=DSP System Toolbox
  Normalization2 : dspmathops/Normalization  NormType=2-norm  Bias=1e-10  NormOver=Each column  Dimension=1  roundingMode=Floor  overflowMode=off  accumDataTypeStr=Inherit: Same as product output  accumLastDataTypeStr=Inherit: Same as product output  outputDataTypeStr=Inherit: Same as product output  outputMin=[]  outputMax=[]  outputLastDataTypeStr=Inherit: Same as product output
      settings: SourceProductName=DSP System Toolbox
  Quaternion Normalize : sharedutil/Quaternion Normalize  aMode=aMode
      settings: SourceProductName=Aerospace Blockset  SourceProductBaseCode=AE
  Transpose : Math  Operator=transpose  SaturateOnIntegerOverflow=on
  Transpose1 : Math  Operator=transpose  SaturateOnIntegerOverflow=on
  Transpose2 : Math  Operator=transpose  SaturateOnIntegerOverflow=on
  Vector Concatenate : Concatenate  NumInputs=3  Mode=Multidimensional array
  q_eci2hill : Outport
  wires:
  3x3 Cross Product1/1 -> Transpose2/1
  Normalization2/1 -> 3x3 Cross Product/2
  Normalization1/1 -> 3x3 Cross Product/1, 3x3 Cross Product1/2, Transpose/1
  Transpose1/1 -> Vector Concatenate/3
  Vector Concatenate/1 -> Direction Cosine Matrix to Quaternions/1
  3x3 Cross Product/1 -> Transpose1/1, 3x3 Cross Product1/1
  Transpose2/1 -> Vector Concatenate/2
  Transpose/1 -> Vector Concatenate/1
  In Bus Element2/1 -> Normalization2/1
  In Bus Element1/1 -> Normalization1/1
  Direction Cosine Matrix to Quaternions/1 -> Quaternion Normalize/1
  Quaternion Normalize/1 -> q_eci2hill/1

== system CubeSat_Simulator/GNC Computer/Guidance/Sun Tracking/Attitude Bias ==
  q Input : Inport
  EulerBias : Inport  Port=2
  Quaternion Multiplication : aerolibutil/Quaternion Multiplication
  Quaternion Normalize : sharedutil/Quaternion Normalize  aMode=aMode
      settings: SourceProductName=Aerospace Blockset  SourceProductBaseCode=AE
  Rotation Angles to Quaternions : sharedtransform/Rotation Angles to Quaternions  rotationOrder=ZYX  aMode=aMode
      settings: SourceProductName=Aerospace Blockset  SourceProductBaseCode=AE
  "\tq Output" : Outport
  wires:
  EulerBias/1 -> Rotation Angles to Quaternions/1
  q Input/1 -> Quaternion Multiplication/1
  Rotation Angles to Quaternions/1 -> Quaternion Multiplication/2
  Quaternion Multiplication/1 -> Quaternion Normalize/1
  Quaternion Normalize/1 -> "\tq Output"/1

== system CubeSat_Simulator/GNC Computer/Guidance/Sun Tracking/Compute Sun Frame ==
  FirstRefECI : Inport
  SecondRefECI : Inport  Port=2
  3x3 Cross Product : sharedutil/3x3 Cross Product  aMode=aMode
      settings: SourceProductBaseCode=AE
  3x3 Cross Product1 : sharedutil/3x3 Cross Product  aMode=aMode
      settings: SourceProductBaseCode=AE
  Direction Cosine Matrix to Quaternions : sharedtransform/Direction Cosine Matrix  to Quaternions  aMode=0  action=None  tolerance=eps(2)
      settings: SourceProductName=Aerospace Blockset  SourceProductBaseCode=AE
  Normalization1 : dspmathops/Normalization  NormType=2-norm  Bias=1e-10  NormOver=Each column  Dimension=1  roundingMode=Floor  overflowMode=off  accumDataTypeStr=Inherit: Same as product output  accumLastDataTypeStr=Inherit: Same as product output  outputDataTypeStr=Inherit: Same as product output  outputMin=[]  outputMax=[]  outputLastDataTypeStr=Inherit: Same as product output
      settings: SourceProductName=DSP System Toolbox
  Normalization2 : dspmathops/Normalization  NormType=2-norm  Bias=1e-10  NormOver=Each column  Dimension=1  roundingMode=Floor  overflowMode=off  accumDataTypeStr=Inherit: Same as product output  accumLastDataTypeStr=Inherit: Same as product output  outputDataTypeStr=Inherit: Same as product output  outputMin=[]  outputMax=[]  outputLastDataTypeStr=Inherit: Same as product output
      settings: SourceProductName=DSP System Toolbox
  Quaternion Normalize : sharedutil/Quaternion Normalize  aMode=aMode
      settings: SourceProductName=Aerospace Blockset  SourceProductBaseCode=AE
  Transpose : Math  Operator=transpose  SaturateOnIntegerOverflow=on
  Transpose1 : Math  Operator=transpose  SaturateOnIntegerOverflow=on
  Transpose2 : Math  Operator=transpose  SaturateOnIntegerOverflow=on
  Vector Concatenate : Concatenate  NumInputs=3  Mode=Multidimensional array
  q_eci2sun : Outport
  wires:
  Transpose2/1 -> Vector Concatenate/2
  3x3 Cross Product/1 -> 3x3 Cross Product1/2, Transpose2/1
  Transpose/1 -> Vector Concatenate/1
  Normalization1/1 -> 3x3 Cross Product/2, 3x3 Cross Product1/1, Transpose/1
  Normalization2/1 -> 3x3 Cross Product/1
  Direction Cosine Matrix to Quaternions/1 -> Quaternion Normalize/1
  Transpose1/1 -> Vector Concatenate/3
  Vector Concatenate/1 -> Direction Cosine Matrix to Quaternions/1
  3x3 Cross Product1/1 -> Transpose1/1
  SecondRefECI/1 -> Normalization2/1
  FirstRefECI/1 -> Normalization1/1
  Quaternion Normalize/1 -> q_eci2sun/1

== system CubeSat_Simulator/GNC Computer/Guidance/Target Tracking/Attitude Bias ==
  q Input : Inport
  EulerBias : Inport  Port=2
  Quaternion Multiplication : aerolibutil/Quaternion Multiplication
  Quaternion Normalize : sharedutil/Quaternion Normalize  aMode=aMode
      settings: SourceProductName=Aerospace Blockset  SourceProductBaseCode=AE
  Rotation Angles to Quaternions : sharedtransform/Rotation Angles to Quaternions  rotationOrder=ZYX  aMode=aMode
      settings: SourceProductName=Aerospace Blockset  SourceProductBaseCode=AE
  "\tq Output" : Outport
  wires:
  EulerBias/1 -> Rotation Angles to Quaternions/1
  q Input/1 -> Quaternion Multiplication/1
  Rotation Angles to Quaternions/1 -> Quaternion Multiplication/2
  Quaternion Multiplication/1 -> Quaternion Normalize/1
  Quaternion Normalize/1 -> "\tq Output"/1

== system CubeSat_Simulator/GNC Computer/Guidance/Target Tracking/Compute Sun Frame ==
  FirstRefECI : Inport
  SecondRefECI : Inport  Port=2
  3x3 Cross Product : sharedutil/3x3 Cross Product  aMode=aMode
      settings: SourceProductBaseCode=AE
  3x3 Cross Product1 : sharedutil/3x3 Cross Product  aMode=aMode
      settings: SourceProductBaseCode=AE
  Direction Cosine Matrix to Quaternions : sharedtransform/Direction Cosine Matrix  to Quaternions  aMode=0  action=None  tolerance=eps(2)
      settings: SourceProductName=Aerospace Blockset  SourceProductBaseCode=AE
  Normalization1 : dspmathops/Normalization  NormType=2-norm  Bias=1e-10  NormOver=Each column  Dimension=1  roundingMode=Floor  overflowMode=off  accumDataTypeStr=Inherit: Same as product output  accumLastDataTypeStr=Inherit: Same as product output  outputDataTypeStr=Inherit: Same as product output  outputMin=[]  outputMax=[]  outputLastDataTypeStr=Inherit: Same as product output
      settings: SourceProductName=DSP System Toolbox
  Normalization2 : dspmathops/Normalization  NormType=2-norm  Bias=1e-10  NormOver=Each column  Dimension=1  roundingMode=Floor  overflowMode=off  accumDataTypeStr=Inherit: Same as product output  accumLastDataTypeStr=Inherit: Same as product output  outputDataTypeStr=Inherit: Same as product output  outputMin=[]  outputMax=[]  outputLastDataTypeStr=Inherit: Same as product output
      settings: SourceProductName=DSP System Toolbox
  Quaternion Normalize : sharedutil/Quaternion Normalize  aMode=aMode
      settings: SourceProductName=Aerospace Blockset  SourceProductBaseCode=AE
  Transpose : Math  Operator=transpose  SaturateOnIntegerOverflow=on
  Transpose1 : Math  Operator=transpose  SaturateOnIntegerOverflow=on
  Transpose2 : Math  Operator=transpose  SaturateOnIntegerOverflow=on
  Vector Concatenate : Concatenate  NumInputs=3  Mode=Multidimensional array
  q_eci2sun : Outport
  wires:
  Transpose2/1 -> Vector Concatenate/2
  3x3 Cross Product/1 -> 3x3 Cross Product1/2, Transpose2/1
  Transpose/1 -> Vector Concatenate/1
  Normalization1/1 -> 3x3 Cross Product/2, 3x3 Cross Product1/1, Transpose/1
  Normalization2/1 -> 3x3 Cross Product/1
  Direction Cosine Matrix to Quaternions/1 -> Quaternion Normalize/1
  Transpose1/1 -> Vector Concatenate/3
  Vector Concatenate/1 -> Direction Cosine Matrix to Quaternions/1
  3x3 Cross Product1/1 -> Transpose1/1
  SecondRefECI/1 -> Normalization2/1
  FirstRefECI/1 -> Normalization1/1
  Quaternion Normalize/1 -> q_eci2sun/1

== system CubeSat_Simulator/GNC Computer/Guidance/Trajectory Planning/Quaternion to Spatial Rotation ==
  q : Inport
  Constant : Constant  Value=[0;0;0]
  Divide : Product  Inputs=*/
  Gain : Gain  Gain=2
  Normalization : dspmathops/Normalization  NormType=Squared 2-norm  Bias=1e-10  NormOver=Each column  Dimension=1  roundingMode=Floor  overflowMode=off  accumDataTypeStr=Inherit: Same as product output  accumLastDataTypeStr=Inherit: Same as product output  outputDataTypeStr=Inherit: Same as product output  outputMin=[]  outputMax=[]  outputLastDataTypeStr=Inherit: Same as product output
      settings: SourceProductName=DSP System Toolbox
  Resolve Division by 0 : Switch  Criteria=u2 ~= 0
  Scalar Part : Selector  InputPortWidth=4  IndexOptions=Index vector (dialog)  Indices=[1]  OutputSizes=1
  Trigonometric Function : Trigonometry  Operator=acos
  Trigonometric Function1 : Trigonometry  OutputSignalType=real
  Vector Part : Selector  InputPortWidth=4  IndexOptions=Index vector (dialog)  Indices=[2 3 4]  OutputSizes=1
  PRA : Outport
  PRV : Outport  Port=2
  wires:
  q/1 -> Scalar Part/1, Vector Part/1
  Scalar Part/1 -> Trigonometric Function/1
  Gain/1 -> PRA/1
  Vector Part/1 -> Divide/1
  Trigonometric Function/1 -> Trigonometric Function1/1, Gain/1
  Trigonometric Function1/1 -> Divide/2, Resolve Division by 0/2
  Normalization/1 -> PRV/1
  Divide/1 -> Resolve Division by 0/1
  Resolve Division by 0/1 -> Normalization/1
  Constant/1 -> Resolve Division by 0/3
